simulink model "nibp_processor_model"  (R2021b)
settings: Solver=VariableStepAuto  StartTime=0.0  StopTime=60  RelTol=1e-3
libraries: Heart_Signal_Processing_Library x2
Description:
  | The Noise Removal Filter works via a cascade of signal processing blocks that work together to clean the signal and sync the pressure waveform
  | and the pump pressure.
  | 
  | The pressure waveform and the pump pressure enters as a time series signal (with a sample time of 0.004 seconds). These signals were parameterized
  | prior to being loaded into Simulink.
  | 
  | The following filters are used on the pressure waveform:
  | 
  | The signals are passed through a bandpass filter. The same bandpass filter from Project 1 which had the tunable pararmeters. For this project the
  | pararneters were tuned as follows: quality factor = 1.5 and center Frequency = 11 Hz. This is done to remove the low frequency baseline in both noisy and
  | noiseless inputs, as well as remove some of the possible high frequency noise in noisy inputs.
  | 
  | Then the signal is passed through a start up buffer that sets the initial bandpass outputs to zero for the first 0.5 seconds, thus avoiding skewing the plot range
  | with the large start up values.
  | 
  | The signal is then cleaned further with a combination of a absolute value filter to remove negative values, and a moving average filter of 38 samples to smooth out the
  | signal.
  | 
  | The signal is then further processed with a gain of 5 to alleveiate some of the attenuation, before placing it through another moving average filter, once again to obtain a smoother curve.
  | 
  | The signal is then squared to help attenuate noise signals that are less than 1 in magnitude, while amplifying the signal values that are larger than one.
  | 
  | The signal is once again amplified by 5 to help alleviate some of the attenuation that occured in the previous step, and placed through a moving average filter to smooth out the curve.
  | 
  | The signal is then placed through a noise threshold where any signal less than 2 in magnitude is considered noise and reduced to zero.
  | 
  | The signal is then passed through a square root filter to reduce the amplification to a more appropriate level now that the noise has been removed.
  | 
  | the signal is then passed through an amplifier of a gain of 1.4 to achieve a signal that is closer in magnitude to the original waveform.
  | 
  | The following filters apply to the pump pressure.
  | 
  | The pump pressure signal is simply delayed by 60 time steps in order to sync with the pressure waveform.
  | 
  | Outputs:
  | 
  | The new clean signals and re-synced are then set as the output.
settings Model: Creator=wallyproenza  LastModifiedBy=wallyproenza

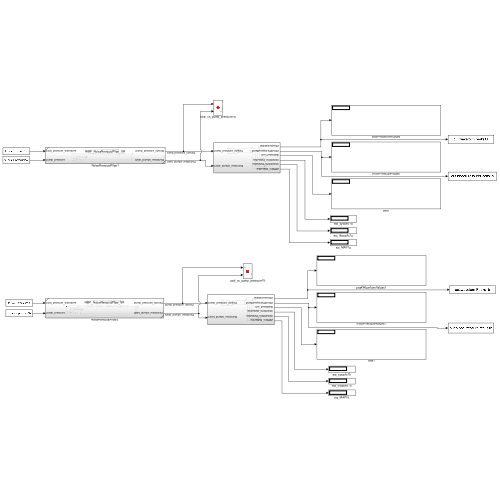
[thumbnail: Simulink's stored preview of the top-level diagram]
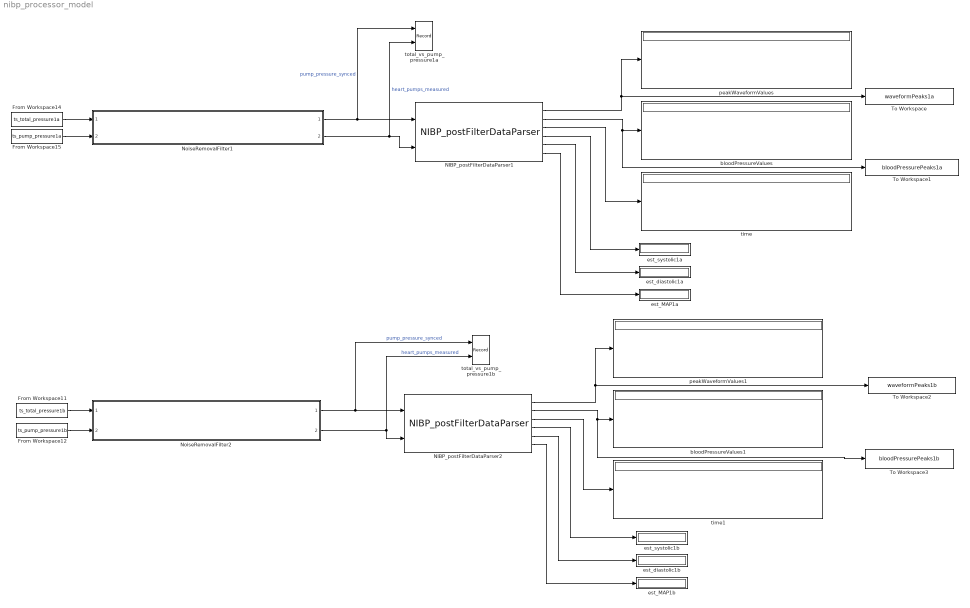
== system nibp_processor_model ==
  From Workspace11 : FromWorkspace  VariableName=ts_total_pressure1b  SampleTime=0.004  OutputAfterFinalValue=Holding final value
  From Workspace12 : FromWorkspace  VariableName=ts_pump_pressure1b  SampleTime=0.004  OutputAfterFinalValue=Holding final value
  From Workspace14 : FromWorkspace  VariableName=ts_total_pressure1a  SampleTime=0.004  OutputAfterFinalValue=Holding final value
  From Workspace15 : FromWorkspace  VariableName=ts_pump_pressure1a  SampleTime=0.004  OutputAfterFinalValue=Holding final value
  NIBP_postFilterDataParser1 : Heart_Signal_Processing_Library/NIBP_postFilterDataParser  SystemSampleTime=-1  VariantActivationTime=update diagram  Latency=0  AutoFrameSizeCalculation=off
  NIBP_postFilterDataParser2 : Heart_Signal_Processing_Library/NIBP_postFilterDataParser  SystemSampleTime=-1  VariantActivationTime=update diagram  Latency=0  AutoFrameSizeCalculation=off
  NoiseRemovalFilter1 : Subsystem  ReferencedSubsystem=NIBP_NoiseRemovalFilter_SR
  NoiseRemovalFilter2 : Subsystem  ReferencedSubsystem=NIBP_NoiseRemovalFilter_SR
  To Workspace : ToWorkspace  VariableName=waveformPeaks1a  SampleTime=-1
      settings: Save2DSignal=2-D array (concatenate along first dimension)
  To Workspace1 : ToWorkspace  VariableName=bloodPressurePeaks1a  SampleTime=-1
      settings: Save2DSignal=2-D array (concatenate along first dimension)
  To Workspace2 : ToWorkspace  VariableName=waveformPeaks1b  SampleTime=-1
      settings: Save2DSignal=2-D array (concatenate along first dimension)
  To Workspace3 : ToWorkspace  VariableName=bloodPressurePeaks1b  SampleTime=-1
      settings: Save2DSignal=2-D array (concatenate along first dimension)
  bloodPressureValues : Display
  bloodPressureValues1 : Display
  est_MAP1a : Display
  est_MAP1b : Display
  est_diastolic1a : Display
  est_diastolic1b : Display
  est_systolic1a : Display
  est_systolic1b : Display
  peakWaveformValues : Display
  peakWaveformValues1 : Display
  time : Display
  time1 : Display
  total_vs_pump_pressure1a : Record  FileSettingsInternal="{\"entries\":[{\"content\":{\"excelSettings\":{\"content\":{},\"type\":\"Streamout.ExcelSettings\"}},\"type\":\"Streamout.FileSettingStorage\",\"uuid\":\"17e9dd7f-06e2-4265-a8b4-4183b2def51a\"}],\"packageUris\":[\"http://schema.mathworks.com/mf0/streamout_blocks/R2020a\"],\"version\":\"1.0\"}"  Layout=[1 1]  SignalsInternal="{\"entries\":[{\"content\":{\"signals\":[{\"content\":{\"blockPath\":[\"nibp_processor_model/total_vs_pump_pressure1a\"],\"channel\":[],\"dimensions\":[1],\"domain\":\"nibp_processor_model/total_vs_pump_pressure1a\",\"lineColor\":\"#a2142f\",\"plots\":[1],\"port\":1,\"sid\":[\"\"],\"signalID\":292,\"signalName\":\"pump_pressure_synced\"},\"type\":\"RecordBlkView.Signal\",\"uuid\":\"6bcdf94a-66c7-4e15-b026-0ca0b3d54f78\"},{\"content\":{\"blockPath\":[\"nibp_processor_model/total_vs_pump_pressure1a\"],\"channel\":[],\"dimensions\":[1],\"domain\":\"nibp_processor_model/total_vs_pump_pressure1a\",\"lineColor\":\"#139fff\",\"plots\":[1],\"port\":2,\"sid\":[\"\"],\"signalID\":296,\"signalName\":\"heart_pumps_measured\"},\"type\":\"RecordBlkView.Signal\",\"uuid\":\"e58309ea-7b2d-413f-bfe2-3a8a0ff24e19\"}]},\"type\":\"RecordBlkView.InputSignals\",\"uuid\":\"a47539bc-7ff8-49ce-b1d6-bc8cb6af9b96\"}],\"packageUris\":[\"http://schema.mathworks.com/mf0/streamout_blocks/R2020a\"],\"version\":\"1.0\"}"  VisualizationBindings="{\"xyplotplugin\":{\"info\":[{\"series\":[{\"bindingParametersList\":[{\"parameter\":\"X-Axis\",\"signalID\":292,\"signalName\":\"pump_pressure_synced\"},{\"parameter\":\"Y-Axis\",\"signalID\":296,\"signalName\":\"heart_pumps_measured\"}],\"seriesID\":3064}],\"subplotID\":1}]}}"  CompatibilityTag=XY  st=-1
  total_vs_pump_pressure1b : Record  FileSettingsInternal="{\"entries\":[{\"content\":{\"excelSettings\":{\"content\":{},\"type\":\"Streamout.ExcelSettings\"}},\"type\":\"Streamout.FileSettingStorage\",\"uuid\":\"e1a465f7-e17b-4f0f-ae27-fe4fdded8e25\"}],\"packageUris\":[\"http://schema.mathworks.com/mf0/streamout_blocks/R2020a\"],\"version\":\"1.0\"}"  Layout=[1 1]  SignalsInternal="{\"entries\":[{\"content\":{\"signals\":[{\"content\":{\"blockPath\":[\"nibp_processor_model/total_vs_pump_pressure1b\"],\"channel\":[],\"dimensions\":[1],\"domain\":\"nibp_processor_model/total_vs_pump_pressure1b\",\"lineColor\":\"#a2142f\",\"plots\":[1],\"port\":1,\"sid\":[\"\"],\"signalID\":284,\"signalName\":\"pump_pressure_synced\"},\"type\":\"RecordBlkView.Signal\",\"uuid\":\"fa2a2a8b-9845-420f-8a27-e00e7067c09b\"},{\"content\":{\"blockPath\":[\"nibp_processor_model/total_vs_pump_pressure1b\"],\"channel\":[],\"dimensions\":[1],\"domain\":\"nibp_processor_model/total_vs_pump_pressure1b\",\"lineColor\":\"#139fff\",\"plots\":[1],\"port\":2,\"sid\":[\"\"],\"signalID\":288,\"signalName\":\"heart_pumps_measured\"},\"type\":\"RecordBlkView.Signal\",\"uuid\":\"ffce9b53-22c8-413b-9c46-d927a8212fbb\"}]},\"type\":\"RecordBlkView.InputSignals\",\"uuid\":\"25e4a94e-a6a9-429d-9b97-a598e6982d69\"}],\"packageUris\":[\"http://schema.mathworks.com/mf0/streamout_blocks/R2020a\"],\"version\":\"1.0\"}"  VisualizationBindings="{\"xyplotplugin\":{\"info\":[{\"series\":[{\"bindingParametersList\":[{\"parameter\":\"X-Axis\",\"signalID\":284,\"signalName\":\"pump_pressure_synced\"},{\"parameter\":\"Y-Axis\",\"signalID\":288,\"signalName\":\"heart_pumps_measured\"}],\"seriesID\":22357}],\"subplotID\":1}]}}"  CompatibilityTag=XY  st=-1
  wires:
  From Workspace14/1 -> NoiseRemovalFilter1/1
  From Workspace15/1 -> NoiseRemovalFilter1/2
  NoiseRemovalFilter1/1 -> NIBP_postFilterDataParser1/1, total_vs_pump_pressure1a/1  "pump_pressure_synced"
  NoiseRemovalFilter1/2 -> NIBP_postFilterDataParser1/2, total_vs_pump_pressure1a/2  "heart_pumps_measured"
  From Workspace11/1 -> NoiseRemovalFilter2/1
  From Workspace12/1 -> NoiseRemovalFilter2/2
  NoiseRemovalFilter2/1 -> total_vs_pump_pressure1b/1, NIBP_postFilterDataParser2/1  "pump_pressure_synced"
  NoiseRemovalFilter2/2 -> total_vs_pump_pressure1b/2, NIBP_postFilterDataParser2/2  "heart_pumps_measured"
  NIBP_postFilterDataParser1/1 -> peakWaveformValues/1, To Workspace/1
  NIBP_postFilterDataParser1/2 -> To Workspace1/1, bloodPressureValues/1
  NIBP_postFilterDataParser1/3 -> time/1
  NIBP_postFilterDataParser1/4 -> est_systolic1a/1
  NIBP_postFilterDataParser1/5 -> est_diastolic1a/1
  NIBP_postFilterDataParser1/6 -> est_MAP1a/1
  NIBP_postFilterDataParser2/2 -> To Workspace3/1, bloodPressureValues1/1
  NIBP_postFilterDataParser2/1 -> peakWaveformValues1/1, To Workspace2/1
  NIBP_postFilterDataParser2/3 -> time1/1
  NIBP_postFilterDataParser2/4 -> est_systolic1b/1
  NIBP_postFilterDataParser2/5 -> est_diastolic1b/1
  NIBP_postFilterDataParser2/6 -> est_MAP1b/1
